simulink model "SomanetTuning"  (R2016b)
settings: Solver=FixedStepDiscrete  StartTime=0.0  StopTime=inf  FixedStep=0.002  RelTol=1e-3  EnableMultiTasking=on
libraries: xpcethercatlib x18, slrtlib x9
(part 2 of 2)

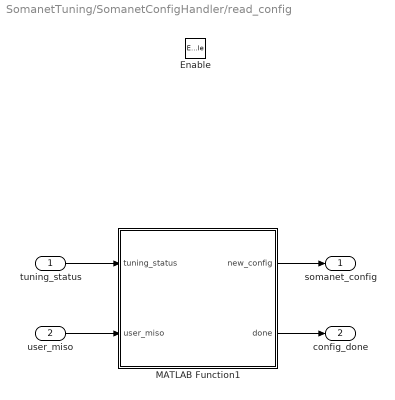
== system SomanetTuning/SomanetConfigHandler/read_config ==
  tuning_status : Inport
  user_miso : Inport  Port=2
  Enable : EnablePort
  MATLAB Function1 : MATLAB Function  TreatAsAtomicUnit=on
  somanet_config : Outport
  config_done : Outport  Port=2
  wires:
  MATLAB Function1/1(new_config) -> somanet_config/1
  MATLAB Function1/2(done) -> config_done/1
  tuning_status/1 -> MATLAB Function1/1(tuning_status)
  user_miso/1 -> MATLAB Function1/2(user_miso)

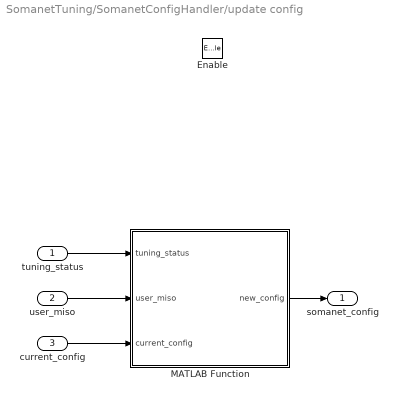
== system SomanetTuning/SomanetConfigHandler/update config ==
  tuning_status : Inport
  user_miso : Inport  Port=2
  current_config : Inport  Port=3
  Enable : EnablePort
  MATLAB Function : MATLAB Function  TreatAsAtomicUnit=on
  somanet_config : Outport
  wires:
  tuning_status/1 -> MATLAB Function/1(tuning_status)
  current_config/1 -> MATLAB Function/3(current_config)
  MATLAB Function/1(new_config) -> somanet_config/1
  user_miso/1 -> MATLAB Function/2(user_miso)

== matlab function SomanetTuning/SetPointGuiHandler/process set point sliders ==
  data: TargetVelocity input; control_strategy output; TargetTorque input; TargetPosition input; TargetPosition output; TargetVelocity output; TargetTorque output; sinus input; omega input
function [control_strategy, TargetPosition,TargetVelocity, TargetTorque] = fcn(TargetVelocity, TargetTorque, TargetPosition, sinus, omega)
    persistent last_V;
    persistent last_T;
    persistent last_P;
    persistent last_mode;
    
    if isempty(last_V)
        last_V = 0;
        last_T = 0;
        last_P = 0;
        last_mode = 0;
    end
    
    if sinus == 0
        omega = 1;
    end

        if TargetVelocity ~= last_V
            last_V = TargetVelocity;
            last_mode = 9;
            control_strategy = 9;
        elseif TargetTorque ~= last_T
            last_T = TargetTorque;
            last_mode = 10;
            control_strategy = 10;
        elseif TargetPosition ~= last_P
            last_P = TargetPosition;
            last_mode = 8;
            control_strategy = 8;
        else
            TargetPosition = omega*last_P;
            TargetVelocity = omega*last_V ;
            TargetTorque = omega*last_T ;
            control_strategy = last_mode;

        end
        
    end

== matlab function SomanetTuning/MATLAB Function ==
  data: state input; is_initializing output; is_updating output
function [is_initializing, is_updating] = enable_subsystems(state)
switch state
    case State.startup
        is_initializing = true;
        is_updating = false;
    case State.tuning
        is_initializing = false;
        is_updating = true;
    otherwise
        is_initializing = false;
        is_updating = false;
end

== stateflow chart SomanetTuning/Chart ==
  state read_config
    entry: state = startup
    exit: state = pending
  state wait_for_somanet
    entry: state = pending
    op_mode_out = int8(0)
  state enter_tuning_mode
    entry: op_mode_out = int8(-128)
  state exit_tuning_mode
    entry: op_mode_out = int8(8)
  state Operational
    entry: state=sync
    exit: last_op_mode = op_mode_somanet
    state=pending
    state Switch_on_disabled
      entry: controlword = 6
      op_mode_out = op_mode_desired
    state Quick_start_active
    state Ready_to_switch_on
      entry: controlword = 7
    state Quick_stop_active_desired
      entry: controlword = 2
    state Operation_enabled
    Quick_start_active -> Switch_on_disabled : [statusword==4160 | statusword==4176 | statusword==4192 | statusword== 4208]
    Switch_on_disabled -> Ready_to_switch_on [order 2] : [op_mode_out ~= -128 && op_mode_somanet == op_mode_out ...
        |  && (statusword==4129 | statusword == 4145) && quick_stop_switch==0]
    Quick_stop_active_desired -> Quick_start_active : [statusword==4103 | statusword == 4119]
    Ready_to_switch_on -> Operation_enabled : [statusword==4135 | statusword == 4151]
    Operation_enabled -> Quick_stop_active_desired : [quick_stop_switch == 1 | op_mode_desired ~= op_mode_out]
  state Fault
    entry: state = fault
    exit: state = pending
    state Fault
    state Fault_remove_desired
      entry: controlword = 128;
    (default) -> Fault.Fault
    Fault.Fault -> Fault_remove_desired : [clear_fault_switch==1]
  note: This block does all state related stuff. By setting
      | flags in different states, simulink blocks outside
      | will be activated and deactivated.
  state SynchronousMode_desired
    entry: op_mode_out = op_mode_desired
  state TuningMode
    entry: state = tuning
    exit: state = pending
  (default) -> wait_for_somanet
  wait_for_somanet -> enter_tuning_mode : [statusword==0]%[statusword==4160 | statusword==4176 | statusword==4192 | statusword== 4208]
  enter_tuning_mode -> read_config : [op_mode_somanet == op_mode_out]
  read_config -> exit_tuning_mode : [reading_config_done == true]
  exit_tuning_mode -> Switch_on_disabled : [op_mode_somanet == op_mode_out]
  Operational -> Fault : [statusword==4136 | statusword == 4104 | statusword == 4120 | statusword == 4152]
  Fault_remove_desired -> Switch_on_disabled : [statusword==4160 | statusword==4176 | statusword==4192 | statusword== 4208]
  SynchronousMode_desired -> Switch_on_disabled : [op_mode_somanet == op_mode_out]
  Switch_on_disabled -> TuningMode [order 1] : [op_mode_somanet == -128]
  TuningMode -> SynchronousMode_desired : [op_mode_desired ~= -128]
  data: statusword input uint16; controlword output double; quick_stop_switch input boolean; clear_fault_switch input; op_mode_desired input int8; op_mode_somanet input; op_mode_out output int8; last_op_mode local int8; reading_config_done input; state output Enum: State

== matlab function SomanetTuning/SomanetConfigHandler/read_config/MATLAB Function1 ==
  data: tuning_status input; new_config output int32 size=18; user_miso input; done output
function [new_config,done] = read_config(tuning_status,user_miso)
    persistent calls;
    persistent buffered_config;
    N_params = 18;
    if(isempty(calls))
        calls = 0;
        buffered_config = zeros(N_params,1);
    end
  
    
    status_mux = bitand(bitsra(tuning_status,16),hex2dec('FF'));
   
    if status_mux <= N_params && status_mux >= 1
        calls = calls + 1;
        buffered_config(status_mux) = user_miso;
        %TODO error handling here?
    end
    
    if calls > N_params % we might want to increase this. We have noticed that sometimes an important value like maxpos does not get properly initalized and instead is zero
        done = true;
    else
        done = false;
    end
    
    new_config = to_signed_int32(buffered_config);
    setConstant('position_p_gui', new_config(8));
    setConstant('position_i_gui', new_config(9));
    setConstant('position_d_gui', new_config(10));
    setConstant('velocity_p_gui', new_config(12));
    setConstant('velocity_i_gui', new_config(13));
    setConstant('velocity_d_gui', new_config(14));
    setConstant('min_position_slider', new_config(4));
    setConstant('max_position_slider', new_config(5));
    setConstant('max_torque_slider', new_config(7));
    setConstant('angle_offset_slider', new_config(1));
    setConstant('changemeplease', 72);
end

== matlab function SomanetTuning/SomanetConfigHandler/update config/MATLAB Function ==
  data: tuning_status input; new_config output; user_miso input; current_config input
function new_config = update_config(tuning_status,user_miso,current_config)
    status_mux = bitand(bitsra(tuning_status,16),hex2dec('FF'));
    N_params = 18;
    
    new_config = current_config;
    if status_mux <= N_params
        new_config(status_mux) = to_signed_int32(user_miso);
        %TODO error handling here?
    end

== matlab function SomanetTuning/TuningCommandGenerator/generates ethercat values to tune somanet ==
  data: desired_config input; current_config input; tuning_command output; positioncontrol_type input; tuning_value output; desired_control_strategy input
function [tuning_command,tuning_value] = gen_tuning_command(desired_config,current_config, positioncontrol_type ,desired_control_strategy)
    persistent lookup;
    persistent last_control_strategy;
    persistent last2_control_strategy;
    persistent last_positioncontrol_type;
    persistent has_issued_command;
    persistent command_timeout;
    
    if (isempty(lookup))
        lookup = [hex2dec('A0'),... %
        hex2dec('B0'),... %
        hex2dec('CC'),... %
        hex2dec('CB'),... %
        hex2dec('CA'),... %
        hex2dec('E0'),... % 
        hex2dec('C0') + 0,hex2dec('C0') + 1,hex2dec('C0') + 2,hex2dec('C0') + 3,... %
        hex2dec('C6') + 0,hex2dec('C6') + 1,hex2dec('C6') + 2,hex2dec('C6') + 3,... %
        hex2dec('CD')]; %
        last_control_strategy = int8(0);
        last2_control_strategy = int8(0);
        last_positioncontrol_type = int32(0);
        has_issued_command = false;
        command_timeout = 0;
    end
    
    if command_timeout > 0
        tuning_command = int32(0);
        tuning_value = int32(0);
        command_timeout = command_timeout -1;
        return;
    end
    
    if(has_issued_command)
        tuning_command = int32(0); %send Ack to Somanet, so it's ready for the next command
        tuning_value = int32(0);
        has_issued_command = false;
        command_timeout = 10; %% Wait 10 loops, which should be 10 * sampletime = 10 * 0.002 = 0.02
        return
    end
    
    for i=1:size(current_config,1)
        if current_config(i) ~= desired_config(i)
            tuning_command = int32(lookup(i));
            tuning_value = desired_config(i);
            has_issued_command = true;
            return;
        end
    end
    
    if last_control_strategy ~= last2_control_strategy
        last2_control_strategy = last_control_strategy;
        tuning_command = int32(0); %send Ack to Somanet, so it's ready for the next command
        tuning_value = int32(0);
        return;
    end
    
    if desired_control_strategy ~= last_control_strategy || positioncontrol_type ~= last_positioncontrol_type
        last_control_strategy = desired_control_strategy;
        if last_positioncontrol_type ~= positioncontrol_type
            last_positioncontrol_type = positioncontrol_type;
            last2_control_strategy = int8(0); % so an Ack will be sent next loop
        end
        disp(['Sending control command to tuning app: ', desired_control_strategy]);
        tuning_command = int32(desired_control_strategy); % these coincide, nice
        tuning_value = positioncontrol_type; % this value is not used when controlstrategy is not position, so this is fine 
        return;
    end    
    

    tuning_command = int32(0);
    tuning_value = int32(0);
end

== matlab function SomanetTuning/determine_opmode/MATLAB Function ==
  data: control_strategy input; fixed_strategy output
function fixed_strategy = ignore_disable_control(control_strategy)
%% Ignores the 'disable control' command button
% When in tuning mode, one can send a disable control command, 7
% When the desired somanet state is cyclic synchronous, the opmode should
% stay the same when this button is accidentally pressed
% Therefore, the last valid strategy is returned
persistent last_strategy;
if(isempty(last_strategy)) 
    last_strategy = int8(0);
end
if(control_strategy ~= 7)
    fixed_strategy = control_strategy;
    last_strategy = control_strategy;
else
    fixed_strategy = last_strategy;
end

end

== matlab function SomanetTuning/SomanetConfigHandler/MATLAB Function ==
  data: enable_config_update input; selection output
function selection = select_config_loop(enable_config_update)
%% Selects whether to output values from read_config or from update_config
% Once update_config has run once, that config stores the correct values
% So, after going back to cyclic operation from tuning mode, update_config
% outputs the correct config even though it's not running
% Therefore: if enable_config_update was true ever, always pick the values
% from update_config

persistent post_init;
if isempty(post_init)
    post_init = false;
end
post_init = or(post_init, enable_config_update);
selection = post_init;
end
